simulink model "Ex_2_sym"  (R2021b)
settings: Solver=VariableStepAuto  StartTime=0.0  StopTime=10.0  RelTol=1e-3
libraries: simulink x2
settings Model: Creator=Leonardo  LastModifiedBy=Leonardo

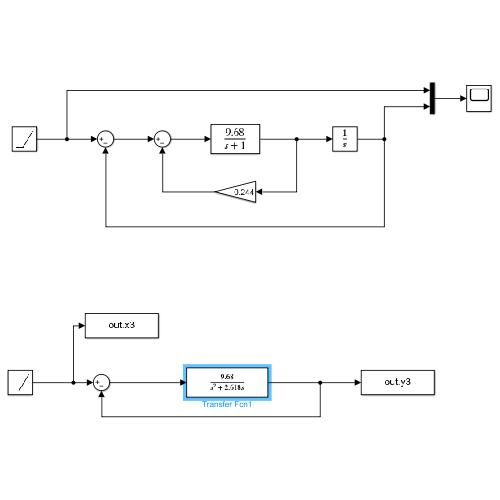
[thumbnail: Simulink's stored preview of the top-level diagram]
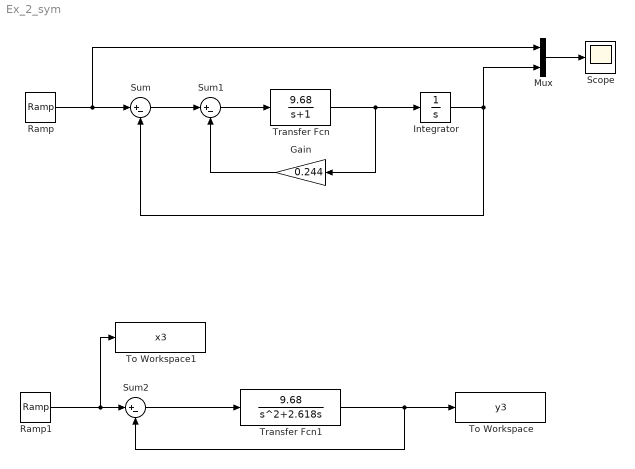
== system Ex_2_sym ==
  Gain : Gain  Gain=0.244
  Integrator : Integrator
  Mux : Mux  Inputs=2
  Ramp : simulink/Sources/Ramp  slope=1  start=0  InitialOutput=0
  Ramp1 : simulink/Sources/Ramp  slope=1  start=0  InitialOutput=0
  Scope : Scope
  Sum : Sum  Inputs=|+-
  Sum1 : Sum  Inputs=|+-
  Sum2 : Sum  Inputs=|+-
  To Workspace : ToWorkspace  VariableName=y3  SaveFormat=Structure With Time  SampleTime=-1
  To Workspace1 : ToWorkspace  VariableName=x3  SaveFormat=Structure With Time  SampleTime=-1
  Transfer Fcn : TransferFcn  Numerator=[9.68]  Denominator=[1 1]
  Transfer Fcn1 : TransferFcn  Numerator=[9.68]  Denominator=[1 2.618 0]
  wires:
  Sum1/1 -> Transfer Fcn/1
  Ramp/1 -> Mux/1, Sum/1
  Ramp1/1 -> To Workspace1/1, Sum2/1
  Sum2/1 -> Transfer Fcn1/1
  Gain/1 -> Sum1/2
  Sum/1 -> Sum1/1
  Transfer Fcn/1 -> Gain/1, Integrator/1
  Transfer Fcn1/1 -> To Workspace/1, Sum2/2
  Mux/1 -> Scope/1
  Integrator/1 -> Mux/2, Sum/2
